simulink model "atan2_cordic"  (R2018b)
settings: Solver=FixedStepDiscrete  StartTime=0.0  StopTime=50  RelTol=1e-3
libraries: commrandsrc3 x2, dspmathops x1
settings Model: SimulationMode=accelerator  Creator=lbai  LastModifiedBy=lbai
settings OptimizationCC: BlockReduction=off  ConditionallyExecuteInputs=off  DefaultParameterBehavior=Inlined
settings DebuggingCC: AlgebraicLoopMsg=error
settings HardwareCC: ProdBitPerPointer=32  ProdBitPerSizeT=32  ProdBitPerPtrDiffT=32  ProdLargestAtomicFloat=None  ProdIntDivRoundTo=Undefined  ProdEndianess=Unspecified  ProdWordSize=32  ProdHWDeviceType=ASIC/FPGA->ASIC/FPGA  TargetBitPerPointer=64  TargetBitPerSizeT=64  TargetBitPerPtrDiffT=64  TargetLongLongMode=on  TargetIntDivRoundTo=Zero  TargetEndianess=LittleEndian  TargetWordSize=64  TargetHWDeviceType=Custom Processor->MATLAB Host Computer  ProdEqTarget=off

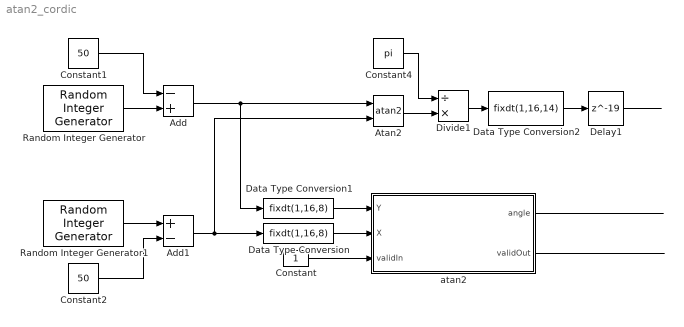
== system atan2_cordic ==
  Add : Sum  Inputs=-+
  Add1 : Sum  Inputs=+-
  Atan2 : Trigonometry  Operator=atan2
  Constant : Constant  OutDataTypeStr=boolean  SampleTime=-1
  Constant1 : Constant  Value=50
  Constant2 : Constant  Value=50
  Constant4 : Constant  Value=pi
  Data Type Conversion : DataTypeConversion  OutDataTypeStr=fixdt(1,16,8)
  Data Type Conversion1 : DataTypeConversion  OutDataTypeStr=fixdt(1,16,8)
  Data Type Conversion2 : DataTypeConversion  OutDataTypeStr=fixdt(1,16,14)
  Delay1 : Delay  DelayLength=19
  Divide1 : Product  Inputs=/*
  Random Integer Generator : commrandsrc3/Random Integer Generator  SetSize=100  SeedSource=Auto  Seed=0  SampleTime=1  SamplesPerFrame=1  OutputDataType=double  SimulateUsing=Interpreted execution
  Random Integer Generator1 : commrandsrc3/Random Integer Generator  SetSize=100  SeedSource=Auto  Seed=0  SampleTime=1  SamplesPerFrame=1  OutputDataType=double  SimulateUsing=Interpreted execution
  atan2 : Subsystem
  wires:
  Constant1/1 -> Add/1
  Random Integer Generator/1 -> Add/2
  Constant2/1 -> Add1/2
  Random Integer Generator1/1 -> Add1/1
  Add/1 -> Atan2/1, Data Type Conversion1/1
  Add1/1 -> Data Type Conversion/1, Atan2/2
  Data Type Conversion1/1 -> atan2/1(Y)
  Data Type Conversion/1 -> atan2/2(X)
  Constant/1 -> atan2/3(validIn)
  atan2/1(angle) -> ?
  Delay1/1 -> ?
  Divide1/1 -> Data Type Conversion2/1
  Constant4/1 -> Divide1/1
  Atan2/1 -> Divide1/2
  Data Type Conversion2/1 -> Delay1/1
  atan2/2(validOut) -> ?

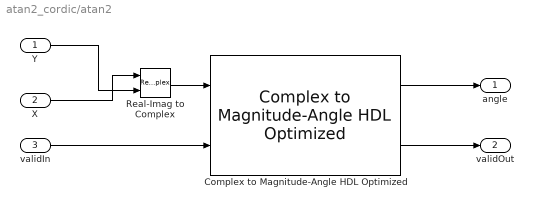
== system atan2_cordic/atan2 ==
  Y : Inport
  X : Inport  Port=2
  validIn : Inport  Port=3
  Complex to Magnitude-Angle HDL Optimized : dspmathops/Complex to Magnitude-Angle HDL Optimized  NumIterationsSource=Auto  NumIterations=10  OutputFormat=Angle  AngleFormat=Normalized  ScaleOutput=on  SimulateUsing=Code generation
      settings: SourceProductName=DSP System Toolbox  SourceProductBaseCode=DS
  Real-Imag to Complex : RealImagToComplex
  angle : Outport
  validOut : Outport  Port=2
  wires:
  Y/1 -> Real-Imag to Complex/2
  Real-Imag to Complex/1 -> Complex to Magnitude-Angle HDL Optimized/1
  validIn/1 -> Complex to Magnitude-Angle HDL Optimized/2
  Complex to Magnitude-Angle HDL Optimized/2 -> validOut/1
  X/1 -> Real-Imag to Complex/1
  Complex to Magnitude-Angle HDL Optimized/1 -> angle/1
